simulink model "Galvo_proto_Cdisc_PT1cont_cc_v63"  (R2013a)
settings: Solver=ode45  StartTime=0.0  StopTime=5e-3  FixedStep=FS  MaxStep=1e-6  RelTol=1e-3  AbsTol=1e-5
PreLoadFcn:
  | vname=@(x) inputname(1);
  | paramCtrl=evalin('base','paramCtrl;');
  | I_LIM=str2num(paramCtrl.I_LIM);
  | Kbc=str2num(paramCtrl.Kbc);
  | FS=evalin('base','FS;');
InitFcn:
  | I_LIM=str2num(paramCtrl.I_LIM);
  | Kbc=str2num(paramCtrl.Kbc);
  | %FS=evalin('base','FS;');
  | 
  | %%%%%%  set scope time range
  | T_STOP=str2num(get_param(gcs,'StopTime'));
  | if numel(T_STOP) > 1
  |    T_STOP=T_STOP(2);
  | else
  |    T_STOP=T_STOP(1);
  | end
  | T_STOP=num2str(T_STOP);
  | 
  | %%%%%%  set scope time range in system @init_callback_fct
  | T_STOP=num2str(str2num(get_param(gcs,'StopTime')));
  | 
  | childs = allchild(0);
  | sol=strfind(upper(get(allchild(0),'Tag')),'VIEWER_PARAMETERS');
  | 
  | if iscell(sol)
  |    ind=find(~cellfun(@isempty, strfind(upper(get(allchild(0),'Tag')),'VIEWER_PARAMETERS')));
  | else
  |    ind=sol;
  | end
  | %ind=find(~cellfun(@isempty, {strfind(upper(get(allchild(0),'Tag')),'VIEWER_PARAMETERS'),[]}))
  | if ~isempty(ind)
  |     set_param(getfield(get(childs(ind),'UserData'),'block'),'TimeRange',T_STOP);
  |     get_param(getfield(get(childs(ind),'UserData'),'block'),'TimeRange');
  | else
  |     warning(sprintf('VIEWER_PARAMETERS object not found\nOpen the config dialog by hand for the first sim start'))
  | end
StartFcn:
  | I_LIM=str2num(paramCtrl.I_LIM);
  | Kbc=str2num(paramCtrl.Kbc);
  | %FS=evalin('base','FS;');
  | 
  | I_LIM
  | Lc
  | Rc
  | Rsh
  | CMG
undefined symbols (not defined in the file or in its folder): CMG, Lc, Rc, Rsh
libraries: simulink x4, simulink_extras x1, dspsigops x1
settings Model: BufferReuse=off  Creator=mainster  LastModifiedBy=mainster
settings SolverCC: AutoInsertRateTranBlk=on
settings DataIOCC: LimitDataPoints=off  SaveOutput=off  SaveTime=off
settings OptimizationCC: BlockReduction=off  OptimizeBlockIOStorage=off  BufferReuse=off  ExpressionFolding=off  LocalBlockOutputs=off
settings ModelReferenceCC: ModelReferenceNumInstancesAllowed=Single

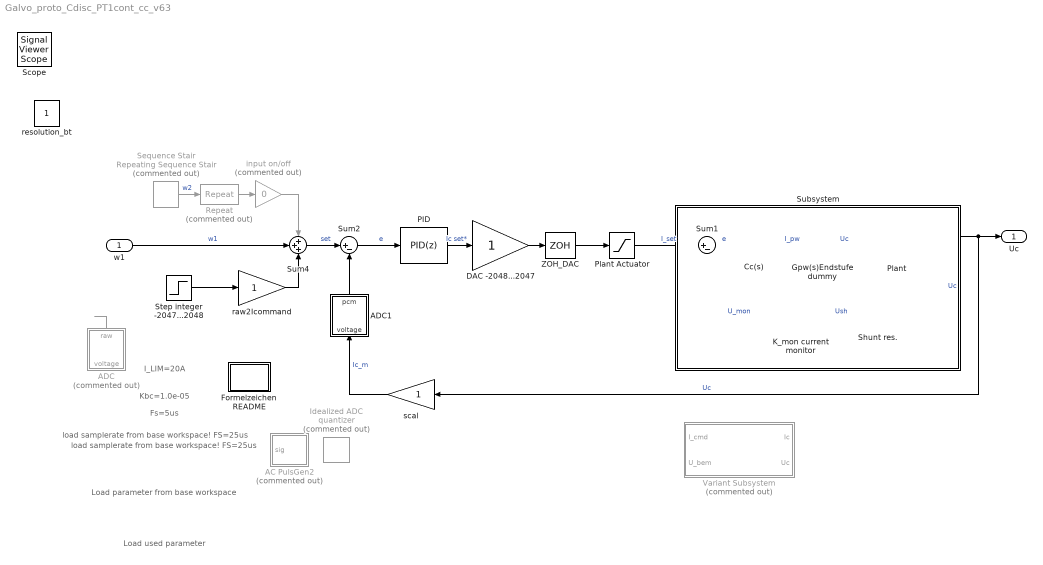
== system Galvo_proto_Cdisc_PT1cont_cc_v63 ==
  note: I_LIM=20A
  note: Kbc=1.0e-05
  note: load samplerate from
      | base workspace!
      | FS=25us
  note: Load parameter from
      | base workspace
  note: Fs=5us
  note: load samplerate from
      | base workspace!
      | FS=25us
  note: Load used parameter
  w1 : Inport  SampleTime=FS
  AC PulsGen2 : Subsystem  Commented=on  mask{sigp=1, sigpp=0, offs=0}
      mask prompts: sigp "Insert signal peak"; sigpp "or signal peak-to-peak"; offs "Insert DC offset"
      mask TypeOptions sigp: PulsGen/Amplitude
      mask Callback sigp:
      | %sigp=get_param([gcb '/PulsGen'],'Amplitude')
      | %SigVal=2*sigp
      mask TypeOptions offs: offset/Value
      mask Display:
      | %str=sprintf('%s',get(gcbh,'ModelName'));
      | port_label('output', 1, '','texmode','off')
      | %text(.05,.98,['{\fontsize{12}\it\bf' strrep(str,'_',' ') '}'],'horizontalAlignment','left','verticalAlignment','top','texmode','on')
      | %text(.5,0.95,['{\fontsize{8}A_{peak}=}'],'horizontalAlignment','center','verticalAlignment','top','texmode','on')
      | disp(sprintf('Up=%.3g\nDC=%.3g',sigp, offs))
      | %disp(['Upp=' sigpp])%, offs))
      | %sprintf('sigpp==%s',sigpp)
      | %text(.15,.05,['{\fontsize{10}\itmechanics}'],'horizontalAlignment','left','verticalAlignment','bottom','texmode','on')
  ADC : Subsystem  Commented=on  mask{bypassVal=-1, resol=12, pass=off}
      mask prompts: resol "resolution [bit]"; pass "bypass ADC"
      mask init:
      | bypass=0;
      mask TypeOptions resol: exp/Value
      mask Callback pass:
      | if strcmpi( get_param(gcb,'pass'),'on')
      |     bypassVal=1;
      | else
      |     bypassVal=0;
      | end
      mask Display:
      | %fprintf('ADC\nGain=%s\n=%i',...
      | %    get_param([gcb '/scale'], 'Gain'),...
      | %    eval( get_param([gcb '/scale'], 'Gain') ));
      | %if bypass
      | 
      | if pass
      |     color('red')
      |     fprintf('bypass\nADC')
      | else
      |     color('black')
      |     fprintf('%i-Bit\nADC',resol)
      | end
  ADC1 : Subsystem  mask{bypass=off}
      mask prompts: bypass "bypass adc"
      mask Callback bypass: %Simulink.Block.eval([gcb '/switch']);
      mask Display:
      | %fprintf('ADC\nGain=%s\n=%i',...
      | %    get_param([gcb '/scale'], 'Gain'),...
      | %    eval( get_param([gcb '/scale'], 'Gain') ));
      | if bypass
      |     color('red')
      |     fprintf('bypass\nADC')
      | else
      |     color('black')
      |     fprintf('ADC')
      | end
  Cc(s) : simulink/Continuous/PID Controller  Controller=P  TimeDomain=Continuous-time  SampleTime=-1  IntegratorMethod=Forward Euler  FilterMethod=Forward Euler  Form=Ideal  P=0.10070221046823  I=1985.39023021624  D=0  N=100  InitialConditionSource=internal  InitialConditionForIntegrator=0  InitialConditionForFilter=0  ExternalReset=none  LimitOutput=on  UpperSaturationLimit=20  LowerSaturationLimit=-20  LinearizeAsGain=on  AntiWindupMode=none  Kb=1  TrackingMode=off  Kt=1  PParamMin=[]  PParamMax=[]  IParamMin=[]  IParamMax=[]  DParamMin=[]  DParamMax=[]  NParamMin=[]  NParamMax=[]  KbParamMin=[]  KbParamMax=[]  KtParamMin=[]  KtParamMax=[]  POutMin=[]  POutMax=[]  IOutMin=[]  IOutMax=[]  DOutMin=[]  DOutMax=[]  NOutMin=[]  NOutMax=[]  KbOutMin=[]  KbOutMax=[]  KtOutMin=[]  KtOutMax=[]  IntegratorOutMin=[]  IntegratorOutMax=[]  FilterOutMin=[]  FilterOutMax=[]  SumOutMin=[]  SumOutMax=[]  SumI1OutMin=[]  SumI1OutMax=[]  SumI2OutMin=[]  SumI2OutMax=[]  SumI3OutMin=[]  SumI3OutMax=[]  SumDOutMin=[]  SumDOutMax=[]  SaturationOutMin=[]  SaturationOutMax=[]  IntegratorContinuousStateAttributes=''  IntegratorStateMustResolveToSignalObject=off  IntegratorRTWStateStorageClass=Auto  FilterContinuousStateAttributes=''  FilterStateMustResolveToSignalObject=off  FilterRTWStateStorageClass=Auto
      settings: AttributesFormatString=P = %<P>
  DAC -2048...2047 : Gain  SampleTime=FS
  Formelzeichen README : Subsystem
  Gpw(s)Endstufe dummy : Gain
  Idealized ADC quantizer : simulink_extras/Additional Discrete/Idealized ADC quantizer  Commented=on  NumberOfConverterBits=16  Vmin=-0.5  Vmax=0.5  OutputDataType=int16  OutputNegativeValues=on
  K_mon current monitor : Gain  Gain=CMG
  PID : simulink/Continuous/PID Controller  Controller=PID  TimeDomain=Discrete-time  SampleTime=FS  IntegratorMethod=Forward Euler  FilterMethod=Forward Euler  Form=Ideal  P=4307.49635546069  I=91281.7891669235  D=0  N=100  InitialConditionSource=internal  InitialConditionForIntegrator=0  InitialConditionForFilter=0  ExternalReset=none  IgnoreLimit=on  LimitOutput=on  UpperSaturationLimit=20  LowerSaturationLimit=-20  LinearizeAsGain=off  AntiWindupMode=back-calculation  Kb=0.1  TrackingMode=off  Kt=0  PParamMin=[]  PParamMax=[]  IParamMin=[]  IParamMax=[]  DParamMin=[]  DParamMax=[]  NParamMin=[]  NParamMax=[]  KbParamMin=[]  KbParamMax=[]  KtParamMin=[]  KtParamMax=[]  POutMin=[]  POutMax=[]  IOutMin=[]  IOutMax=[]  DOutMin=[]  DOutMax=[]  NOutMin=[]  NOutMax=[]  KbOutMin=[]  KbOutMax=[]  KtOutMin=[]  KtOutMax=[]  IntegratorOutMin=[]  IntegratorOutMax=[]  FilterOutMin=[]  FilterOutMax=[]  SumOutMin=[]  SumOutMax=[]  SumI1OutMin=[]  SumI1OutMax=[]  SumI2OutMin=[]  SumI2OutMax=[]  SumI3OutMin=[]  SumI3OutMax=[]  SumDOutMin=[]  SumDOutMax=[]  SaturationOutMin=[]  SaturationOutMax=[]  IntegratorContinuousStateAttributes=''  IntegratorStateMustResolveToSignalObject=off  IntegratorRTWStateStorageClass=Auto  FilterContinuousStateAttributes=''  FilterStateMustResolveToSignalObject=off  FilterRTWStateStorageClass=Auto
      settings: AttributesFormatString=AWM=%<AntiWindupMode>\nD=%<D>\nI=%<I>\nN=%<N>\nP=%<P>\nLimit=+-%<UpperSaturationLimit>
  Plant : Subsystem  Variant=on  OverrideUsingVariant=Variant_LR
  Plant Actuator : Saturate  UpperLimit=I_LIM  LowerLimit=-I_LIM  SampleTime=FS
      settings: AttributesFormatString=I_lim+: %<UpperLimit>\nI_lim-: %<LowerLimit>
  Repeat : dspsigops/Repeat  Commented=on  N=length(str2num(get_param([gcs '/Sequence Stair'], 'OutValues')))  InputProcessing=Columns as channels (frame based)  RateOptions=Allow multirate processing  ic=0  mode=Unused parameter value
  Sequence Stair : simulink/Sources/Repeating Sequence Stair  Commented=on  OutValues="pi/180*[-10     0    14     3    12     9     3    -9     6 1 2   -15     5     6     8    14    17].'"  tsamp=(str2num(get_param(gcs,'StopTime')) / length(str2num(get_param([gcs '/Sequence Stair'], 'OutValues'))))  OutMin=[]  OutMax=[]  OutDataTypeStr=double  OutputDataTypeScalingMode=double  OutDataType=fixdt(0,8)  ConRadixGroup=Best Precision: Vector-wise  OutScaling=2^-12
  Shunt res. : Gain
  Step integer -2047...2048 : Step  Time=1e-3  SampleTime=FS  ZeroCross=off
      settings: AttributesFormatString=Ampl.: %<After>\ntime:%<Time>
  Subsystem : Subsystem
      mask Display: text(.05,.90,['{\fontsize{13}\it\bfCurrent Compensator}'],'horizontalAlignment','left','verticalAlignment','bottom','texmode','on')
  Sum1 : Sum  Inputs=|+-
  Sum2 : Sum  Inputs=|+-  SampleTime=FS
  Sum4 : Sum  Inputs=+++  SampleTime=FS
  Variant Subsystem : Subsystem  Commented=on  Variant=on  OverrideUsingVariant=Gv_CCmod
  ZOH_DAC : ZeroOrderHold  SampleTime=FS
  input on/off : Gain  Commented=on  Gain=0  SampleTime=FS
  raw2Icommand : Gain  SampleTime=FS
  scal : Gain  SampleTime=FS
  Uc : Outport  SampleTime=FS
  Scope : SignalViewerScope  IOType=viewer  NumInputPorts=7  LegendLocations=|  RefreshTime=0.033391
      | 0.86298     0.93763    0.099588    0.037818
      | 0.82246     0.78623      0.1408    0.037818
      | 0.83001     0.65035    0.083104    0.021231
      | 0.83001     0.51553     0.13255    0.021231
      | 0.85474     0.39729     0.20673    0.037818
      | 0.85474     0.26247    0.091346    0.021231
      |       0           0           0           0
      settings: ShowLegends=on  TimeRange=0.025  YMin=0~0~-2~0~0~0~-5  YMax=5~7~5~20~20~0.15~5
  resolution_bt : Constant  IOType=siggen
  wires:
  w1/1 -> Sum4/2  "w1"
  PID/1 -> DAC -2048...2047/1  "Ic set*"
  Plant Actuator/1 -> Sum1/1  "I_set"
  Sequence Stair/1 -> Repeat/1  "w2"
  Repeat/1 -> input on/off/1
  Sum2/1 -> PID/1  "e"
  Sum4/1 -> Sum2/1  "set"
  Step integer -2047...2048/1 -> raw2Icommand/1
  input on/off/1 -> Sum4/1
  raw2Icommand/1 -> Sum4/3
  ZOH_DAC/1 -> Plant Actuator/1
  ADC/1(raw) -> ?
  ADC1/1(pcm) -> Sum2/2
  scal/1 -> ADC1/1(voltage)  "Ic_m"
  Sum1/1 -> Cc(s)/1  "e"
  Cc(s)/1 -> Gpw(s)Endstufe dummy/1  "I_pw"
  K_mon current monitor/1 -> Sum1/2  "U_mon"
  Shunt res./1 -> K_mon current monitor/1  "Ush"
  Gpw(s)Endstufe dummy/1 -> Plant/1(U_c)  "Uc"
  Plant/2(Ic) -> Shunt res./1  "Uc"
  Plant/1(Uout) -> scal/1, Uc/1  "Uc"
  DAC -2048...2047/1 -> ZOH_DAC/1

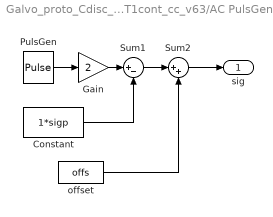
== system Galvo_proto_Cdisc_PT1cont_cc_v63/AC PulsGen2 ==
  Constant : Constant  Value=1*sigp
  Gain : Gain  Gain=2
  PulsGen : DiscretePulseGenerator  PulseType=Time based  Amplitude=sigp  Period=4e-3  PulseWidth=50  PhaseDelay=0.5e-3  SampleTime=FS
      settings: AttributesFormatString=A=%<Amplitude>\nPeri=%<Period>
  Sum1 : Sum  Inputs=|+-
  Sum2 : Sum  Inputs=|++
  offset : Constant  Value=offs
  sig : Outport
  wires:
  Sum2/1 -> sig/1
  PulsGen/1 -> Gain/1
  offset/1 -> Sum2/2
  Gain/1 -> Sum1/1
  Sum1/1 -> Sum2/1
  Constant/1 -> Sum1/2

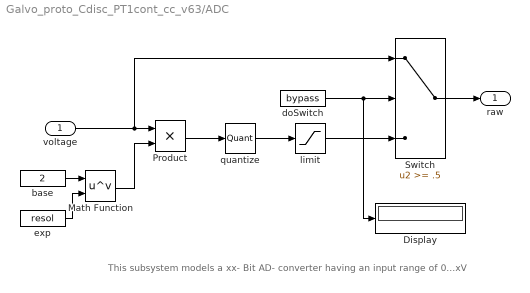
== system Galvo_proto_Cdisc_PT1cont_cc_v63/ADC ==
  note: This subsystem models a xx- Bit AD- converter
      | having an input  range of 0...xV
  voltage : Inport
  Display : Display
  Math Function : Math  Operator=pow  SaturateOnIntegerOverflow=on
  Product : Product
  Switch : Switch  Threshold=.5
  base : Constant  Value=2
  doSwitch : Constant  Value=bypass
  exp : Constant  Value=resol
  limit : Saturate  UpperLimit=2^11-1  LowerLimit=-2^11
      settings: AttributesFormatString=hiLim: %<UpperLimit>\nlowLim: %<LowerLimit>
  quantize : Quantizer
  raw : Outport
  wires:
  limit/1 -> Switch/3
  quantize/1 -> limit/1
  doSwitch/1 -> Display/1, Switch/2
  Switch/1 -> raw/1
  base/1 -> Math Function/1
  exp/1 -> Math Function/2
  voltage/1 -> Switch/1, Product/1
  Math Function/1 -> Product/2
  Product/1 -> quantize/1

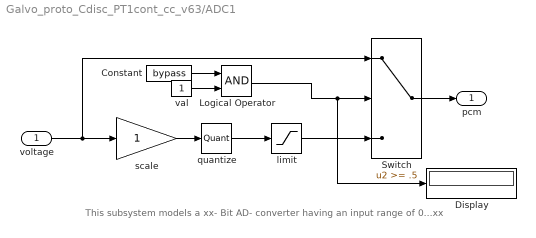
== system Galvo_proto_Cdisc_PT1cont_cc_v63/ADC1 ==
  note: This subsystem models a xx- Bit AD- converter
      | having an input  range of 0...xx
  voltage : Inport
  Constant : Constant  Value=bypass
  Display : Display
  Logical Operator : Logic  AllPortsSameDT=off  OutDataTypeStr=boolean
  Switch : Switch  Threshold=.5
  limit : Saturate  UpperLimit=2^11-1  LowerLimit=-2^11
      settings: AttributesFormatString=%<LowerLimit>\n%<UpperLimit>
  quantize : Quantizer
  scale : Gain  SaturateOnIntegerOverflow=on  OutDataTypeStr=Inherit: Same as input  ParamDataTypeStr=Inherit: Same as input
  val : Constant
  pcm : Outport
  wires:
  limit/1 -> Switch/3
  scale/1 -> quantize/1
  quantize/1 -> limit/1
  voltage/1 -> Switch/1, scale/1
  Switch/1 -> pcm/1
  val/1 -> Logical Operator/2
  Constant/1 -> Logical Operator/1
  Logical Operator/1 -> Display/1, Switch/2

== system Galvo_proto_Cdisc_PT1cont_cc_v63/Formelzeichen README ==
  note: Te: 		electrical torque, gen. by coils		[Nm]
      |  Ic: 			coil current							[A]
      |  Tfr:		rotor dynamic friction torque 		[Nm]
      |  Trb:		torsion bar torque					[Nm]
      |  Tw:		angular momentum				[Nm*s]
      |  w:			angular velocity 					[rad/s]
      |  yrad:		angular position 					[rad]
      |  ydeg:		angular position 					[°]
      |  Ucci:		current controller input				[V]
      |  Ucco:		current controller output			[V]
      |  Ush:		shunt voltage						[V]
  note: L_{c  }	coil inductance 							[H]
      |  R_{c  }	coil resistance							[\Omega]
      |  R_{SH }	current shunt resistance				[\Omega]
      |  J_{R  }	rotor inertia 							[kg*m²]
      |  K_{TB }	torsion bar torque const. 			[Nm/rad]
      |  K_{BM }	back EMF const.							[V*s/rad]
      |  K_{FR }	rotor dyn. friction torque const.	[Nm*s/rad]
      |  K_{MT }	el. magnetic torque const.			[Nm/A]
  note: balance of force: 	Te=Ttb+Tfr
      | 					Te - (Ttb+Tfr)=0  ->  no movement
      |
      |  integrate( 1 Nm )dt = 1 Nm*s
      |  (Nm*s)(kg*m²)⁻¹ = (N*s/kg)*m⁻¹ = m/(s*m) = rad
  note: prototyp v1.3
      | 20-04-2015
      |
      | Signal + Power PCB
      | Allgemeine überprüfung des Regleralgorithmus anhand
      | einer PT1 Strecke (RC-Glied)
      | Parametrierung des diskreten PID Galvo Qt Gui während Laufzeit

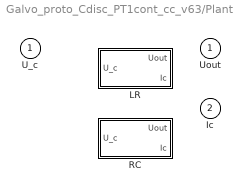
== system Galvo_proto_Cdisc_PT1cont_cc_v63/Plant ==
  U_c : Inport
  LR : Subsystem  VariantControl=Variant_LR
  RC : Subsystem  VariantControl=Variant_RC
  Uout : Outport
  Ic : Outport  Port=2

== system Galvo_proto_Cdisc_PT1cont_cc_v63/Subsystem ==

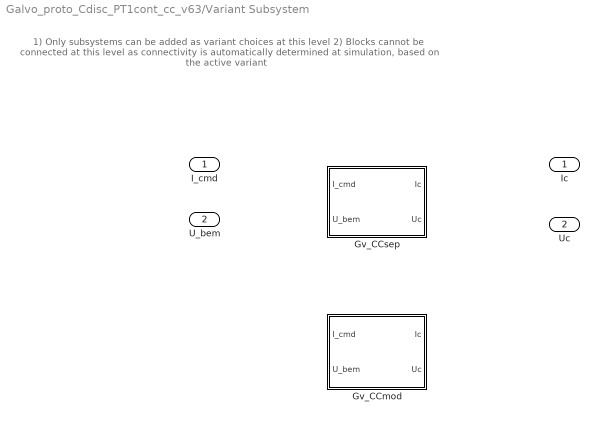
== system Galvo_proto_Cdisc_PT1cont_cc_v63/Variant Subsystem ==
  note: 1) Only subsystems can be added as variant choices at this level
      | 2) Blocks cannot be connected at this level as connectivity is
      | automatically determined at simulation, based on the active variant
  I_cmd : Inport
  U_bem : Inport  Port=2
  Gv_CCmod : Subsystem  VariantControl=Gv_CCmod
  Gv_CCsep : Subsystem  VariantControl=Gv_CCsep
  Ic : Outport  SampleTime=FS
  Uc : Outport  Port=2  SampleTime=FS

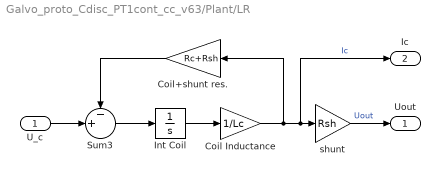
== system Galvo_proto_Cdisc_PT1cont_cc_v63/Plant/LR ==
  U_c : Inport
  Coil Inductance : Gain  Gain=1/Lc
  Coil+shunt res. : Gain  Gain=Rc+Rsh
  Int Coil : Integrator
  Sum3 : Sum  Inputs=-+|
  shunt : Gain  Gain=Rsh
  Uout : Outport
  Ic : Outport  Port=2
  wires:
  U_c/1 -> Sum3/2
  Int Coil/1 -> Coil Inductance/1
  Coil+shunt res./1 -> Sum3/1
  Sum3/1 -> Int Coil/1
  Coil Inductance/1 -> Coil+shunt res./1, Ic/1, shunt/1  "Ic"
  shunt/1 -> Uout/1  "Uout"

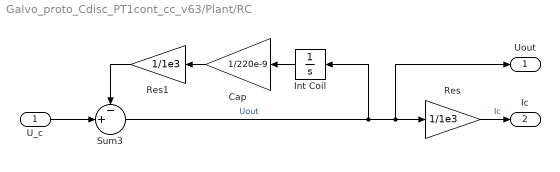
== system Galvo_proto_Cdisc_PT1cont_cc_v63/Plant/RC ==
  U_c : Inport
  Cap : Gain  Gain=1/220e-9
  Int Coil : Integrator
  Res : Gain  Gain=1/1e3
  Res1 : Gain  Gain=1/1e3
  Sum3 : Sum  Inputs=-+|
  Uout : Outport
  Ic : Outport  Port=2
  wires:
  U_c/1 -> Sum3/2
  Int Coil/1 -> Cap/1
  Cap/1 -> Res1/1
  Sum3/1 -> Res/1, Uout/1, Int Coil/1  "Uout"
  Res/1 -> Ic/1  "Ic"
  Res1/1 -> Sum3/1

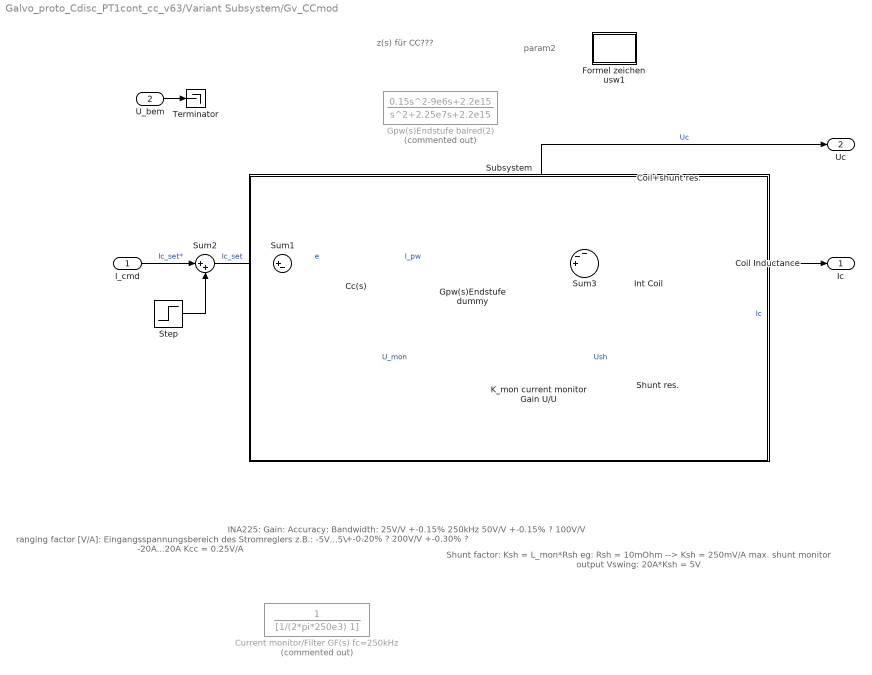
== system Galvo_proto_Cdisc_PT1cont_cc_v63/Variant Subsystem/Gv_CCmod ==
  note: z(s) für
      | CC???
  note: ranging factor [V/A]:
      | Eingangsspannungsbereich des
      | Stromreglers z.B.:
      | -5V...5V --> -20A...20A
      | Kcc = 0.25V/A
  note: Shunt factor:
      | Ksh = L_mon*Rsh
      |
      | eg: Rsh = 10mOhm
      |
      | --> Ksh = 250mV/A
      | max. shunt monitor
      | output Vswing:
      | 20A*Ksh = 5V
  note: INA225:
      | Gain:		Accuracy:		Bandwidth:
      | 25V/V		+-0.15%		250kHz
      | 50V/V		+-0.15%		?
      | 100V/V	+-0.20%		?
      | 200V/V	+-0.30%		?
  note: param2
  I_cmd : Inport  SampleTime=FS
  U_bem : Inport  Port=2  SampleTime=FS
  Cc(s) : simulink/Continuous/PID Controller  Controller=P  TimeDomain=Continuous-time  SampleTime=-1  IntegratorMethod=Forward Euler  FilterMethod=Forward Euler  Form=Ideal  P=15.5227390982487  I=1985.39023021624  D=0  N=100  InitialConditionSource=internal  InitialConditionForIntegrator=0  InitialConditionForFilter=0  ExternalReset=none  LimitOutput=off  UpperSaturationLimit=inf  LowerSaturationLimit=-inf  LinearizeAsGain=on  AntiWindupMode=none  Kb=1  TrackingMode=off  Kt=1  PParamMin=[]  PParamMax=[]  IParamMin=[]  IParamMax=[]  DParamMin=[]  DParamMax=[]  NParamMin=[]  NParamMax=[]  KbParamMin=[]  KbParamMax=[]  KtParamMin=[]  KtParamMax=[]  POutMin=[]  POutMax=[]  IOutMin=[]  IOutMax=[]  DOutMin=[]  DOutMax=[]  NOutMin=[]  NOutMax=[]  KbOutMin=[]  KbOutMax=[]  KtOutMin=[]  KtOutMax=[]  IntegratorOutMin=[]  IntegratorOutMax=[]  FilterOutMin=[]  FilterOutMax=[]  SumOutMin=[]  SumOutMax=[]  SumI1OutMin=[]  SumI1OutMax=[]  SumI2OutMin=[]  SumI2OutMax=[]  SumI3OutMin=[]  SumI3OutMax=[]  SumDOutMin=[]  SumDOutMax=[]  SaturationOutMin=[]  SaturationOutMax=[]  IntegratorContinuousStateAttributes=''  IntegratorStateMustResolveToSignalObject=off  IntegratorRTWStateStorageClass=Auto  FilterContinuousStateAttributes=''  FilterStateMustResolveToSignalObject=off  FilterRTWStateStorageClass=Auto
      settings: AttributesFormatString=P = %<P>
  Coil Inductance : Gain  Gain=1/Lc
  Coil+shunt res. : Gain  Gain=Rc+Rsh
  Current monitor/Filter GF(s) fc=250kHz : TransferFcn  Commented=on  Denominator=[1/(2*pi*250e3) 1]
  Formel zeichen usw1 : Subsystem
  Gpw(s)Endstufe balred(2) : TransferFcn  Commented=on  Numerator=[0.15 -9e6 2.2e15]  Denominator=[1 2.25e7 2.2e15]
  Gpw(s)Endstufe dummy : Gain
  Int Coil : Integrator
  K_mon current monitor Gain U/U : Gain  Gain=1/Rsh
  Shunt res. : Gain  Gain=Rsh
  Step : Step  Time=0  After=0
      settings: AttributesFormatString=%<Time>
  Subsystem : Subsystem
      mask Display: text(.05,.90,['{\fontsize{13}\it\bfCurrent Compensator}'],'horizontalAlignment','left','verticalAlignment','bottom','texmode','on')
  Sum1 : Sum  Inputs=|+-
  Sum2 : Sum  Inputs=|++
  Sum3 : Sum  Inputs=--+||
  Terminator : Terminator
  Ic : Outport  SampleTime=FS
  Uc : Outport  Port=2  SampleTime=FS
  wires:
  I_cmd/1 -> Sum2/1  "Ic_set*"
  Sum1/1 -> Cc(s)/1  "e"
  Sum3/1 -> Int Coil/1
  Int Coil/1 -> Coil Inductance/1
  Cc(s)/1 -> Gpw(s)Endstufe dummy/1  "I_pw"
  K_mon current monitor Gain U/U/1 -> Sum1/2  "U_mon"
  Shunt res./1 -> K_mon current monitor Gain U/U/1  "Ush"
  Gpw(s)Endstufe dummy/1 -> Uc/1, Sum3/3  "Uc"
  Coil+shunt res./1 -> Sum3/1
  Sum2/1 -> Sum1/1  "Ic_set"
  Step/1 -> Sum2/2
  Coil Inductance/1 -> Ic/1, Coil+shunt res./1, Shunt res./1  "Ic"
  U_bem/1 -> Terminator/1

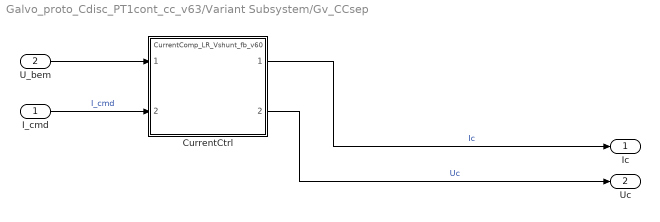
== system Galvo_proto_Cdisc_PT1cont_cc_v63/Variant Subsystem/Gv_CCsep ==
  I_cmd : Inport  SampleTime=FS
  U_bem : Inport  Port=2  SampleTime=FS
  CurrentCtrl : ModelReference  ModelNameDialog=CurrentComp_LR_Vshunt_fb_v60.slx  SimulationMode=Normal  Variant=on  OverrideUsingVariant=cc_v20  ModelReferenceVersion=1.94  CopyOfModelName=CurrentComp_LR_Vshunt_fb_v60.slx  DefaultDataLogging=on
      mask Display:
      | str=sprintf('%s',get(gcbh,'ModelName'));
      | port_label('input', 2, 'I_{Set}','texmode','on')
      | color('red');
      | port_label('input', 1, 'U_{BEM}','texmode','on')
      | color('black');
      | port_label('output', 1, 'I_{Coil}','texmode','on')
      | port_label('output', 2, 'U_{Coil}','texmode','on')
      | %text(.05,.98,['{\fontsize{12}\it\bf' strrep(str,'_',' ') '}'],'horizontalAlignment','left','verticalAlignment','top','texmode','on')
      | text(.5,0.95,['{\fontsize{12}\it\bfG_{cc}(s)}'],'horizontalAlignment','center','verticalAlignment','top','texmode','on')
      | %text(.15,.05,['{\fontsize{10}\itmechanics}'],'horizontalAlignment','left','verticalAlignment','bottom','texmode','on')
  Ic : Outport  SampleTime=FS
  Uc : Outport  Port=2  SampleTime=FS
  wires:
  CurrentCtrl/1 -> Ic/1  "Ic"
  I_cmd/1 -> CurrentCtrl/2  "I_cmd"
  CurrentCtrl/2 -> Uc/1  "Uc"
  U_bem/1 -> CurrentCtrl/1

== system Galvo_proto_Cdisc_PT1cont_cc_v63/Variant Subsystem/Gv_CCmod/Formel zeichen usw1 ==
  note: Te: 		electrical torque, gen. by coils		[Nm]
      |  Ic: 			coil current							[A]
      |  Tfr:		rotor dynamic friction torque 		[Nm]
      |  Trb:		torsion bar torque					[Nm]
      |  Tw:		angular momentum				[Nm*s]
      |  w:			angular velocity 					[rad/s]
      |  yrad:		angular position 					[rad]
      |  ydeg:		angular position 					[°]
      |  Ucci:		current controller input				[V]
      |  Ucco:		current controller output			[V]
      |  Ush:		shunt voltage						[V]
  note: L_{c  }	coil inductance 							[H]
      |  R_{c  }	coil resistance							[\Omega]
      |  R_{SH }	current shunt resistance				[\Omega]
      |  J_{R  }	rotor inertia 							[kg*m²]
      |  K_{TB }	torsion bar torque const. 			[Nm/rad]
      |  K_{BM }	back EMF const.							[V*s/rad]
      |  K_{FR }	rotor dyn. friction torque const.	[Nm*s/rad]
      |  K_{MT }	el. magnetic torque const.			[Nm/A]
  note: balance of force: 	Te=Ttb+Tfr
      | 					Te - (Ttb+Tfr)=0  ->  no movement
      |
      |  integrate( 1 Nm )dt = 1 Nm*s
      |  (Nm*s)(kg*m²)⁻¹ = (N*s/kg)*m⁻¹ = m/(s*m) = rad

== system Galvo_proto_Cdisc_PT1cont_cc_v63/Variant Subsystem/Gv_CCmod/Subsystem ==
